simulink model "Task3"  (R2022a)
settings: Solver=FixedStepAuto  StartTime=0.0  StopTime=10  FixedStep=0.0001  RelTol=1e-3
undefined symbols (not defined in the file): a2, a3, k1, k2, s1, s2, T
libraries: simulink x1
settings Model: Creator=Family  LastModifiedBy=Family

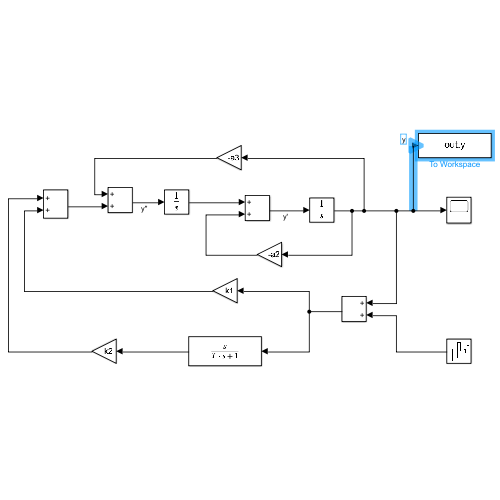
[thumbnail: Simulink's stored preview of the top-level diagram]
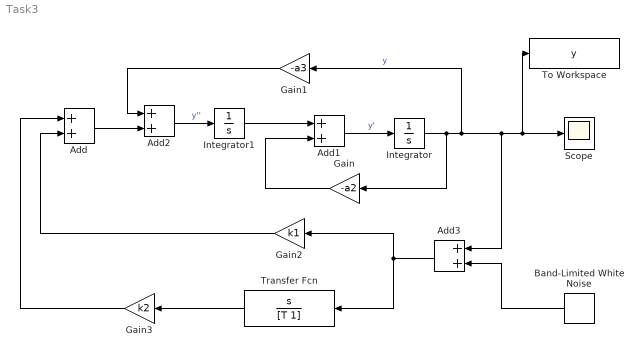
== system Task3 ==
  Add{,1..3} (4 alike) : Sum
  Band-Limited White Noise : simulink/Sources/Band-Limited White Noise  Cov=[0.01]  Ts=0.01  seed=[23341]
  Gain : Gain  Gain=-a2
  Gain1 : Gain  Gain=-a3
  Gain2 : Gain  Gain=k1
  Gain3 : Gain  Gain=k2
  Integrator : Integrator  InitialCondition=s1
  Integrator1 : Integrator  InitialCondition=s2
  Scope : Scope
  To Workspace : ToWorkspace  VariableName=y  SaveFormat=Timeseries  SampleTime=-1
  Transfer Fcn : TransferFcn  Numerator=[1 0]  Denominator=[T 1]
  wires:
  Integrator/1 -> Gain/1, Gain1/1, Scope/1, To Workspace/1, Add3/1  "y"
  Transfer Fcn/1 -> Gain3/1
  Add1/1 -> Integrator/1  "y'"
  Gain/1 -> Add1/2
  Integrator1/1 -> Add1/1
  Add2/1 -> Integrator1/1  "y''"
  Gain1/1 -> Add2/1
  Add/1 -> Add2/2
  Gain2/1 -> Add/2
  Gain3/1 -> Add/1
  Band-Limited White Noise/1 -> Add3/2
  Add3/1 -> Gain2/1, Transfer Fcn/1
